simulink model "tpe_2_2"  (R2022b)
settings: Solver=VariableStepAuto  StartTime=0.0  StopTime=10.0  RelTol=1e-3
InitFcn:
  | %Parameters
  | b1 = 15; b2 = 30; M1 = 5; M2 = 20;
  | 
  | %Matrixes
  | A = [0, 0, 1, 0; 0, 0, 0, 1; -(k1+k2)/M1, k2/M1, -(b1+b2)/M1, b2/M1; k2/M2, -k2/M2, b2/M2, -b2/M2];
  | B = [0 0;0 0;1/M1 0;0 1/M2];
  | C = eye(4);
  | C34 = C(3:4,:);
  | Ke = [-5 0; 0 -20];
settings Model: Creator=garci  LastModifiedBy=garci

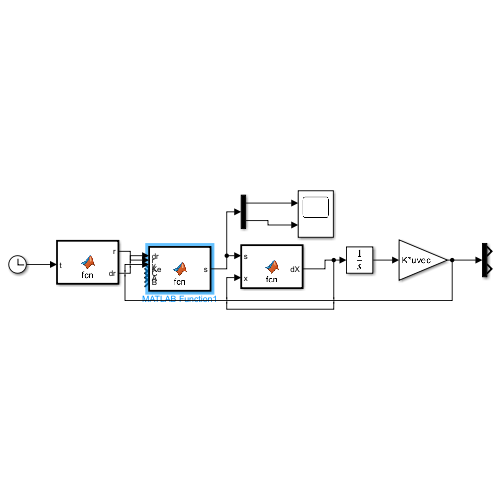
[thumbnail: Simulink's stored preview of the top-level diagram]
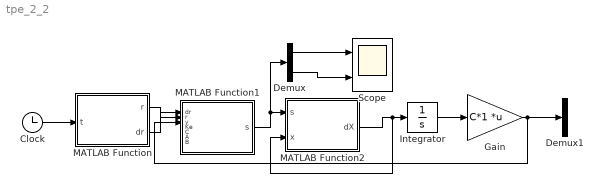
== system tpe_2_2 ==
  Clock : Clock
  Demux : Demux  Outputs=2
  Demux1 : Demux  Outputs=2
  Gain : Gain  Gain=C*1  Multiplication=Matrix(K*u) (u vector)
  Integrator : Integrator
  MATLAB Function : MATLAB Function  TreatAsAtomicUnit=on
  MATLAB Function1 : MATLAB Function  TreatAsAtomicUnit=on
  MATLAB Function2 : MATLAB Function  TreatAsAtomicUnit=on
  Scope : Scope  NumInputPorts=2
  wires:
  Integrator/1 -> Gain/1
  MATLAB Function2/1(dX) -> MATLAB Function2/2(x), Integrator/1
  MATLAB Function1/1(s) -> Demux/1, MATLAB Function2/1(s)
  MATLAB Function/1(r) -> MATLAB Function1/2(r)
  MATLAB Function/2(dr) -> MATLAB Function1/1(dr)
  Gain/1 -> MATLAB Function1/3(y), Demux1/1
  Demux/1 -> Scope/1
  Demux/2 -> Scope/2
  Clock/1 -> MATLAB Function/1(t)

== matlab function tpe_2_2/MATLAB Function1 ==
  data: dr input; r input; s output; y input; Ke input; C input; A input; B input
function s  = fcn(dr, r, y, Ke, C, A, B)

    X = y;
    C34 = C((3:4),:);
    y4 = C34*X; 
    e = r - y4;
    s = (C34*B)^-1*(dr - C34*A*X - Ke*e);

== matlab function tpe_2_2/MATLAB Function ==
  data: t input; r output; dr output
function [r, dr] = fcn(t)

r1 = cos(t).^2; 
dr1 = -2*cos(t).*sin(t);
r2 = sin(t); 
dr2 = cos(t);
r = [r1;r2]; 
dr = [dr1;dr2];

== matlab function tpe_2_2/MATLAB Function2 ==
  data: s input; dX output; x input
function dX  = fcn(s,x)

dX = 1;
